simulink model "s_ident3"  (Simulink 4.00)
settings: Solver=ode45  StartTime=0.0  StopTime=100  RelTol=1e-3
libraries: slident x1
settings Model: LastModifiedBy=Administrator  BlockReductionOpt=off

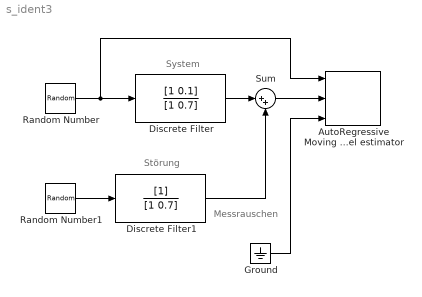
== system s_ident3 ==
  note: Messrauschen
  note: System
  note: Störung
  AutoRegressive Moving Average with eXternal input model estimator : slident/AutoRegressive Moving Average with eXternal input model estimator  MaskParam1=512  MaskParam2=[1 2 1 0]  MaskParam3=64  MaskParam4=0.1
  Discrete Filter : DiscreteFilter  Numerator=[1 0.1]  Denominator=[1 0.7]  SampleTime=0.1  Realization=auto
  Discrete Filter1 : DiscreteFilter  Numerator=[1]  Denominator=[1 0.7]  SampleTime=0.1  Realization=auto
  Ground : Ground
  Random Number : RandomNumber  Mean=0  Variance=1  Seed=0  SampleTime=0.1
  Random Number1 : RandomNumber  Mean=0  Variance=1  Seed=1479  SampleTime=0.1
  Sum : Sum  Inputs=|++  SaturateOnIntegerOverflow=on
  wires:
  Random Number/1 -> Discrete Filter/1, AutoRegressive Moving Average with eXternal input model estimator/1
  Random Number1/1 -> Discrete Filter1/1
  Discrete Filter/1 -> Sum/1
  Sum/1 -> AutoRegressive Moving Average with eXternal input model estimator/2
  Discrete Filter1/1 -> Sum/2
  Ground/1 -> AutoRegressive Moving Average with eXternal input model estimator/3
